simulink model "transformer_test"  (R2016a)
settings: Solver=VariableStepAuto  StartTime=0.0  StopTime=10.0  RelTol=1e-3
libraries: simulink x1
settings Model: Creator=ja  LastModifiedBy=ja

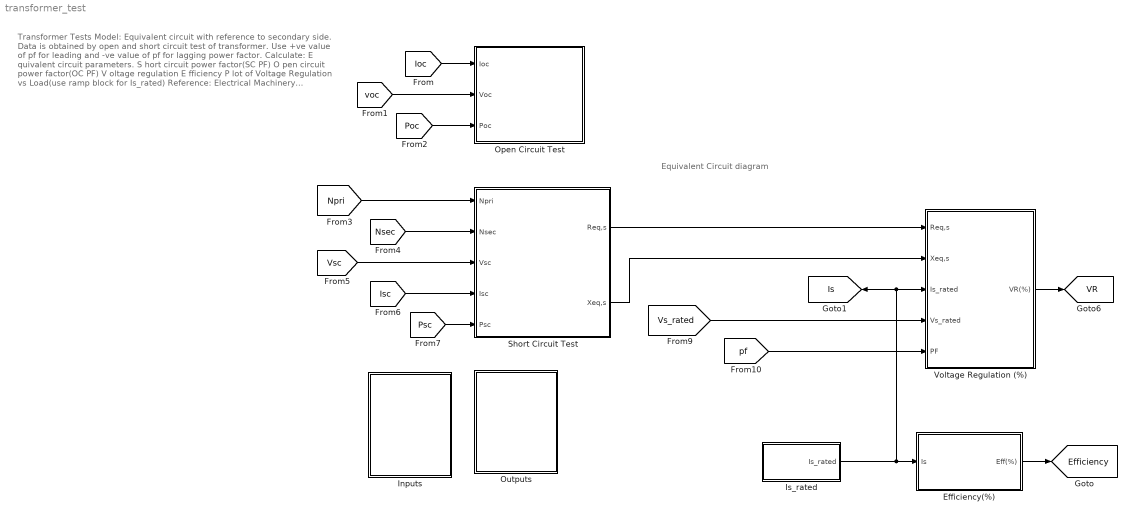
== system transformer_test ==
  note: Equivalent Circuit diagram
  note: Transformer Tests Model:
      | Equivalent circuit with reference to secondary side.
      | Data is obtained by open and short circuit test of transformer.
      | Use +ve value of pf for leading and -ve value of pf for lagging power factor.
      | Calculate:
      | E quivalent circuit parameters.
      | S hort circuit power factor(SC PF)
      | O pen circuit power factor(OC PF)
      | V oltage regulation
      | E fficiency
      | P lot of Voltage Regulation vs Load(use ramp block for Is_rated)
      |
      | Reference:
      | Electrical Machinery Fundamentals by Stephen J. Chapman.
      | (Example 2-5)
  Efficiency(%) : Subsystem
  Inputs : Subsystem
  Is_rated : Subsystem
  Open Circuit Test : Subsystem
  Outputs : Subsystem
  Short Circuit Test : Subsystem
  Voltage Regulation (%) : Subsystem
  tag scope: Efficiency=global, Is=global, VR=global
  wires:
  [Ioc] -> Open Circuit Test/1(Ioc)
  [voc] -> Open Circuit Test/2(Voc)
  [Poc] -> Open Circuit Test/3(Poc)
  [Vsc] -> Short Circuit Test/3(Vsc)
  [Isc] -> Short Circuit Test/4(Isc)
  [Psc] -> Short Circuit Test/5(Psc)
  Short Circuit Test/1(Req,s) -> Voltage Regulation (%)/1(Req,s)
  Short Circuit Test/2(Xeq,s) -> Voltage Regulation (%)/2(Xeq,s)
  [Npri] -> Short Circuit Test/1(Npri)
  [Nsec] -> Short Circuit Test/2(Nsec)
  [Vs_rated] -> Voltage Regulation (%)/4(Vs_rated)
  [pf] -> Voltage Regulation (%)/5(PF)
  Voltage Regulation (%)/1(VR(%)) -> [VR]
  Efficiency(%)/1(Eff(%)) -> [Efficiency]
  Is_rated/1(Is_rated) -> Voltage Regulation (%)/3(Is_rated), [Is], Efficiency(%)/1(Is)

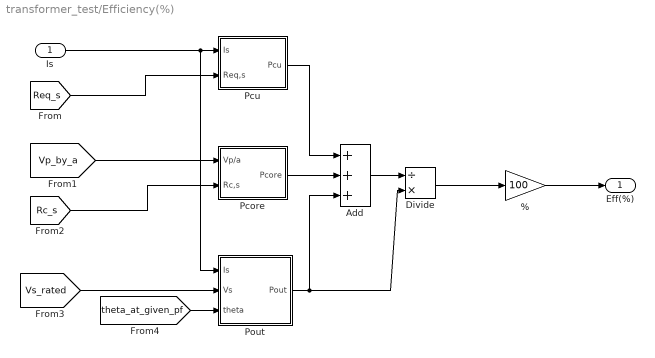
== system transformer_test/Efficiency(%) ==
  Is : Inport
  % : Gain  Gain=100
  Add : Sum  Inputs=+++
  Divide : Product  Inputs=/*
  Pcore : Subsystem
  Pcu : Subsystem
  Pout : Subsystem
  Eff(%) : Outport
  wires:
  Is/1 -> Pout/1(Is), Pcu/1(Is)
  [Req_s] -> Pcu/2(Req,s)
  [Vp_by_a] -> Pcore/1(Vp/a)
  [Rc_s] -> Pcore/2(Rc,s)
  [Vs_rated] -> Pout/2(Vs)
  [theta_at_given_pf] -> Pout/3(theta)
  Pcu/1(Pcu) -> Add/1
  Pcore/1(Pcore) -> Add/2
  Pout/1(Pout) -> Divide/2, Add/3
  Add/1 -> Divide/1
  Divide/1 -> %/1
  %/1 -> Eff(%)/1

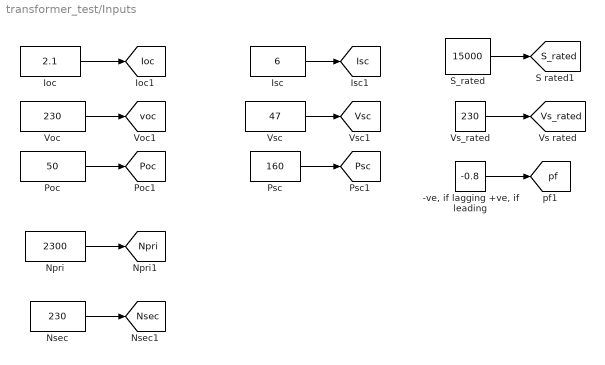
== system transformer_test/Inputs ==
  "-ve, if lagging +ve, if leading" : Constant  Value=-0.8
  Ioc : Constant  Value=2.1
  Isc : Constant  Value=6
  Npri : Constant  Value=2300
  Nsec : Constant  Value=230
  Poc : Constant  Value=50
  Psc : Constant  Value=160
  S_rated : Constant  Value=15000
  Voc : Constant  Value=230
  Vs_rated : Constant  Value=230
  Vsc : Constant  Value=47
  tag scope: Ioc=global, Isc=global, Npri=global, Nsec=global, Poc=global, Psc=global, S_rated=global, Vs_rated=global, Vsc=global, pf=global, voc=global
  wires:
  S_rated/1 -> [S_rated]
  Ioc/1 -> [Ioc]
  Isc/1 -> [Isc]
  Nsec/1 -> [Nsec]
  Voc/1 -> [voc]
  Poc/1 -> [Poc]
  Vsc/1 -> [Vsc]
  Npri/1 -> [Npri]
  Vs_rated/1 -> [Vs_rated]
  Psc/1 -> [Psc]
  "-ve, if lagging +ve, if leading"/1 -> [pf]

== system transformer_test/Is_rated ==
  Is,rated(full load Current on Sec) : Product  Inputs=/*
  Is_rated : Outport
  wires:
  Is,rated(full load Current on Sec)/1 -> Is_rated/1
  [S_rated] -> Is,rated(full load Current on Sec)/2
  [Vs_rated] -> Is,rated(full load Current on Sec)/1

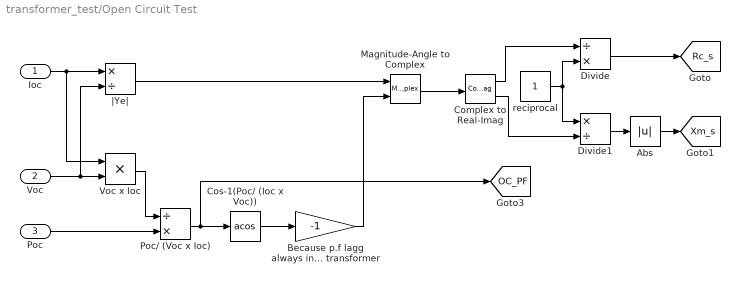
== system transformer_test/Open Circuit Test ==
  Ioc : Inport
  Voc : Inport  Port=2
  Poc : Inport  Port=3
  Abs : Abs
  "Because p.f lagg always in transformer " : Gain  Gain=-1
  Complex to Real-Imag : ComplexToRealImag
  Cos-1(Poc/ (Ioc x Voc)) : Trigonometry  Operator=acos
  Divide : Product  Inputs=/*
  Divide1 : Product  Inputs=*/
  Magnitude-Angle to Complex : MagnitudeAngleToComplex
  Poc/ (Voc x Ioc) : Product  Inputs=/*
  Voc x Ioc : Product
  reciprocal : Constant
  |Ye| : Product  Inputs=*/
  tag scope: OC_PF=global, Rc_s=global, Xm_s=global
  wires:
  Ioc/1 -> |Ye|/1, Voc x Ioc/1
  Complex to Real-Imag/1 -> Divide/1
  reciprocal/1 -> Divide1/1, Divide/2
  Divide/1 -> [Rc_s]
  Poc/ (Voc x Ioc)/1 -> Cos-1(Poc/ (Ioc x Voc))/1, [OC_PF]
  "Because p.f lagg always in transformer "/1 -> Magnitude-Angle to Complex/2
  Complex to Real-Imag/2 -> Divide1/2
  Voc x Ioc/1 -> Poc/ (Voc x Ioc)/1
  Voc/1 -> Voc x Ioc/2, |Ye|/2
  Magnitude-Angle to Complex/1 -> Complex to Real-Imag/1
  Cos-1(Poc/ (Ioc x Voc))/1 -> "Because p.f lagg always in transformer "/1
  |Ye|/1 -> Magnitude-Angle to Complex/1
  Poc/1 -> Poc/ (Voc x Ioc)/2
  Divide1/1 -> Abs/1
  Abs/1 -> [Xm_s]

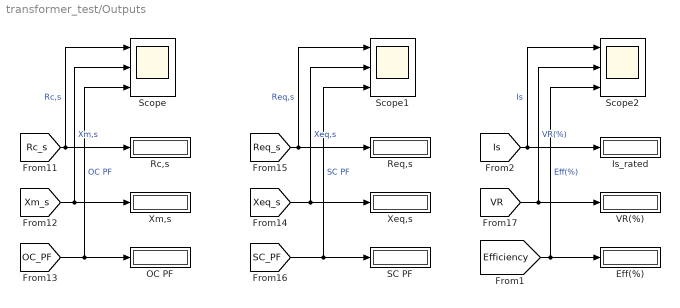
== system transformer_test/Outputs ==
  Eff(%) : Display
  Is_rated : Display
  OC PF : Display
  Rc,s : Display
  Req,s : Display
  SC PF : Display
  Scope : Scope  NumInputPorts=3
  Scope1 : Scope  NumInputPorts=3
  Scope2 : Scope  NumInputPorts=3
  VR(%) : Display
  Xeq,s : Display
  Xm,s : Display
  wires:
  [VR] -> VR(%)/1, Scope2/2  "VR(%)"
  [Rc_s] -> Scope/1, Rc,s/1  "Rc,s"
  [Xm_s] -> Scope/2, Xm,s/1  "Xm,s"
  [Xeq_s] -> Scope1/2, Xeq,s/1  "Xeq,s"
  [Req_s] -> Req,s/1, Scope1/1  "Req,s"
  [SC_PF] -> Scope1/3, SC PF/1  "SC PF"
  [Efficiency] -> Eff(%)/1, Scope2/3  "Eff(%)"
  [OC_PF] -> Scope/3, OC PF/1  "OC PF"
  [Is] -> Is_rated/1, Scope2/1  "Is"

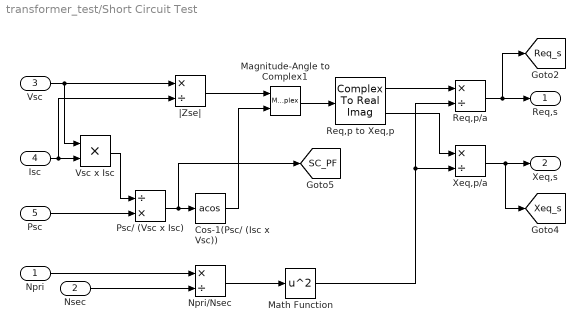
== system transformer_test/Short Circuit Test ==
  Npri : Inport
  Nsec : Inport  Port=2
  Vsc : Inport  Port=3
  Isc : Inport  Port=4
  Psc : Inport  Port=5
  Cos-1(Psc/ (Isc x Vsc)) : Trigonometry  Operator=acos
  Magnitude-Angle to Complex1 : MagnitudeAngleToComplex
  Math Function : Math  Operator=square  SaturateOnIntegerOverflow=on
  Npri/Nsec : Product  Inputs=*/
  Psc/ (Vsc x Isc) : Product  Inputs=/*
  Req,p to Xeq,p : ComplexToRealImag
  Req,p/a : Product  Inputs=*/
  Vsc x Isc : Product
  Xeq,p/a : Product  Inputs=*/
  |Zse| : Product  Inputs=*/
  Req,s : Outport
  Xeq,s : Outport  Port=2
  tag scope: Req_s=global, SC_PF=global, Xeq_s=global
  wires:
  Magnitude-Angle to Complex1/1 -> Req,p to Xeq,p/1
  Psc/ (Vsc x Isc)/1 -> Cos-1(Psc/ (Isc x Vsc))/1, [SC_PF]
  |Zse|/1 -> Magnitude-Angle to Complex1/1
  Cos-1(Psc/ (Isc x Vsc))/1 -> Magnitude-Angle to Complex1/2
  Isc/1 -> Vsc x Isc/2, |Zse|/2
  Vsc x Isc/1 -> Psc/ (Vsc x Isc)/1
  Vsc/1 -> |Zse|/1, Vsc x Isc/1
  Psc/1 -> Psc/ (Vsc x Isc)/2
  Npri/1 -> Npri/Nsec/1
  Nsec/1 -> Npri/Nsec/2
  Req,p to Xeq,p/1 -> Req,p/a/1
  Req,p to Xeq,p/2 -> Xeq,p/a/1
  Npri/Nsec/1 -> Math Function/1
  Math Function/1 -> Xeq,p/a/2, Req,p/a/2
  Req,p/a/1 -> [Req_s], Req,s/1
  Xeq,p/a/1 -> [Xeq_s], Xeq,s/1

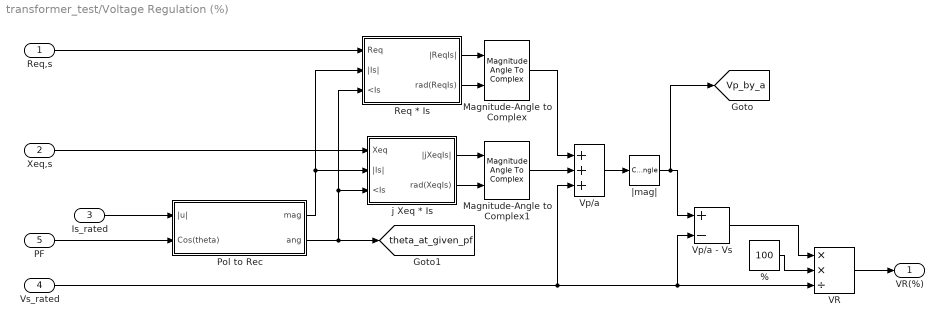
== system transformer_test/Voltage Regulation (%) ==
  Req,s : Inport
  Xeq,s : Inport  Port=2
  Is_rated : Inport  Port=3
  Vs_rated : Inport  Port=4
  PF : Inport  Port=5
  % : Constant  Value=100
  Magnitude-Angle to Complex : MagnitudeAngleToComplex
  Magnitude-Angle to Complex1 : MagnitudeAngleToComplex
  Pol to Rec : Subsystem
  Req * Is : Subsystem
  VR : Product  Inputs=**/
  Vp/a : Sum  Inputs=+++
  Vp/a - Vs : Sum  Inputs=+-
  j Xeq * Is : Subsystem
  |mag| : ComplexToMagnitudeAngle  Output=Magnitude
  VR(%) : Outport
  tag scope: Vp_by_a=global, theta_at_given_pf=global
  wires:
  VR/1 -> VR(%)/1
  Vs_rated/1 -> VR/3, Vp/a - Vs/2, Vp/a/3
  Pol to Rec/1(mag) -> Req * Is/2(|Is|), j Xeq * Is/2(|Is|)
  PF/1 -> Pol to Rec/2(Cos(theta))
  Vp/a/1 -> |mag|/1
  |mag|/1 -> [Vp_by_a], Vp/a - Vs/1
  Req,s/1 -> Req * Is/1(Req)
  Pol to Rec/2(ang) -> [theta_at_given_pf], j Xeq * Is/3(<Is), Req * Is/3(<Is)
  Xeq,s/1 -> j Xeq * Is/1(Xeq)
  Req * Is/1(|ReqIs|) -> Magnitude-Angle to Complex/1
  j Xeq * Is/1(|jXeqIs|) -> Magnitude-Angle to Complex1/1
  j Xeq * Is/2(rad(XeqIs)) -> Magnitude-Angle to Complex1/2
  Req * Is/2(rad(ReqIs)) -> Magnitude-Angle to Complex/2
  Magnitude-Angle to Complex1/1 -> Vp/a/2
  Magnitude-Angle to Complex/1 -> Vp/a/1
  %/1 -> VR/2
  Vp/a - Vs/1 -> VR/1
  Is_rated/1 -> Pol to Rec/1(|u|)

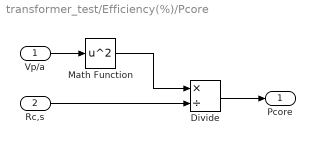
== system transformer_test/Efficiency(%)/Pcore ==
  Vp/a : Inport
  Rc,s : Inport  Port=2
  Divide : Product  Inputs=*/
  Math Function : Math  Operator=square  SaturateOnIntegerOverflow=on
  Pcore : Outport
  wires:
  Divide/1 -> Pcore/1
  Rc,s/1 -> Divide/2
  Math Function/1 -> Divide/1
  Vp/a/1 -> Math Function/1

== system transformer_test/Efficiency(%)/Pcu ==
  Is : Inport
  Req,s : Inport  Port=2
  Math Function : Math  Operator=square  SaturateOnIntegerOverflow=on
  Product : Product
  Pcu : Outport
  wires:
  Is/1 -> Math Function/1
  Math Function/1 -> Product/1
  Req,s/1 -> Product/2
  Product/1 -> Pcu/1

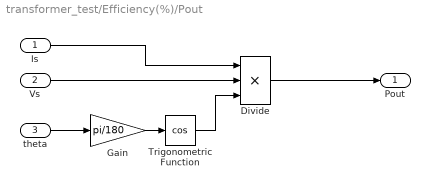
== system transformer_test/Efficiency(%)/Pout ==
  Is : Inport
  Vs : Inport  Port=2
  theta : Inport  Port=3
  Divide : Product  Inputs=***
  Gain : Gain  Gain=pi/180
  Trigonometric Function : Trigonometry  Operator=cos
  Pout : Outport
  wires:
  Is/1 -> Divide/1
  Vs/1 -> Divide/2
  Divide/1 -> Pout/1
  theta/1 -> Gain/1
  Gain/1 -> Trigonometric Function/1
  Trigonometric Function/1 -> Divide/3

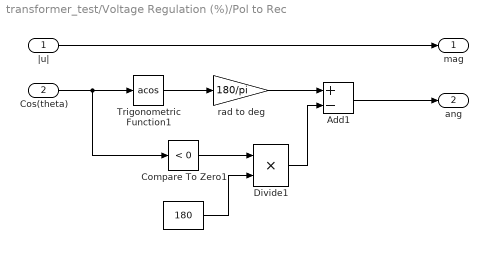
== system transformer_test/Voltage Regulation (%)/Pol to Rec ==
  |u| : Inport
  Cos(theta) : Inport  Port=2
  "  " : Constant  Value=180
  Add1 : Sum  Inputs=+-
  Compare To Zero1 : simulink/Logic and Bit Operations/Compare To Zero  relop=<  OutDataTypeStr=boolean
  Divide1 : Product  Inputs=**
  Trigonometric Function1 : Trigonometry  Operator=acos
  rad to deg : Gain  Gain=180/pi
  mag : Outport
  ang : Outport  Port=2
  wires:
  Cos(theta)/1 -> Trigonometric Function1/1, Compare To Zero1/1
  Trigonometric Function1/1 -> rad to deg/1
  Compare To Zero1/1 -> Divide1/1
  "  "/1 -> Divide1/2
  Divide1/1 -> Add1/2
  Add1/1 -> ang/1
  |u|/1 -> mag/1
  rad to deg/1 -> Add1/1

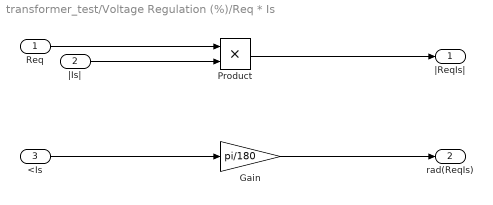
== system transformer_test/Voltage Regulation (%)/Req * Is ==
  Req : Inport
  |Is| : Inport  Port=2
  <Is : Inport  Port=3
  Gain : Gain  Gain=pi/180
  Product : Product
  |ReqIs| : Outport
  rad(ReqIs) : Outport  Port=2
  wires:
  |Is|/1 -> Product/2
  Req/1 -> Product/1
  Product/1 -> |ReqIs|/1
  <Is/1 -> Gain/1
  Gain/1 -> rad(ReqIs)/1

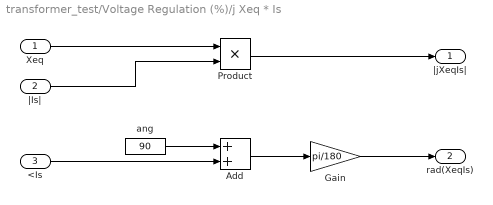
== system transformer_test/Voltage Regulation (%)/j Xeq * Is ==
  Xeq : Inport
  |Is| : Inport  Port=2
  <Is : Inport  Port=3
  Add : Sum
  Gain : Gain  Gain=pi/180
  Product : Product
  ang : Constant  Value=90
  |jXeqIs| : Outport
  rad(XeqIs) : Outport  Port=2
  wires:
  Product/1 -> |jXeqIs|/1
  Xeq/1 -> Product/1
  |Is|/1 -> Product/2
  ang/1 -> Add/1
  <Is/1 -> Add/2
  Add/1 -> Gain/1
  Gain/1 -> rad(XeqIs)/1
